simulink model "Project_Trial1"  (R2023b)
settings: Solver=VariableStepAuto  StartTime=0.0  StopTime=10.0  MaxStep=0.01  RelTol=1e-3
settings Model: Creator=LL  LastModifiedBy=LL

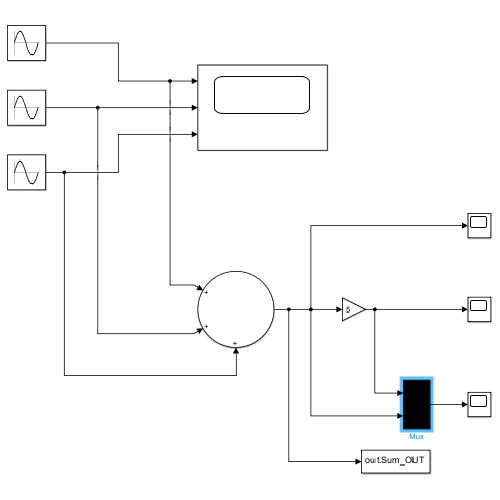
[thumbnail: Simulink's stored preview of the top-level diagram]
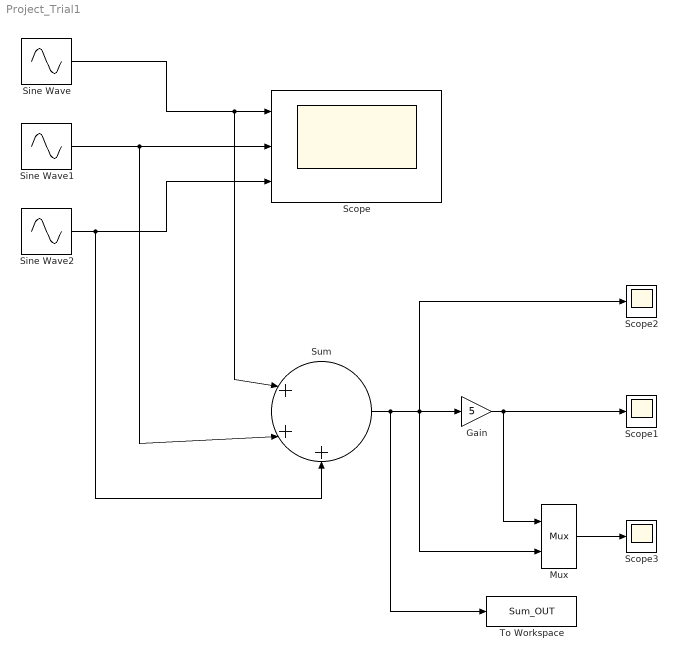
== system Project_Trial1 ==
  Gain : Gain  Gain=5
  Mux : Mux  Inputs=2
  Scope : Scope  NumInputPorts=3
  Scope1 : Scope
  Scope2 : Scope
  Scope3 : Scope
  Sine Wave : Sin  SampleTime=0
  Sine Wave1 : Sin  Frequency=5  SampleTime=0
  Sine Wave2 : Sin  Frequency=10  SampleTime=0
  Sum : Sum  Inputs=|+++
  To Workspace : ToWorkspace  VariableName=Sum_OUT  SaveFormat=Timeseries  SampleTime=-1
  wires:
  Sine Wave1/1 -> Sum/2, Scope/2
  Sine Wave2/1 -> Sum/3, Scope/3
  Sine Wave/1 -> Sum/1, Scope/1
  Sum/1 -> To Workspace/1, Mux/2, Scope2/1, Gain/1
  Gain/1 -> Mux/1, Scope1/1
  Mux/1 -> Scope3/1
